simulink subsystem "Measurements"  (R2022a)
settings: Solver=VariableStepAuto  StartTime=0.0  StopTime=10.0  RelTol=1e-3
undefined symbols (not defined in the file): D0, D1, D13, D3, D6, PTA1, PTC16, PTC17, PTC2, PTD1
libraries: frdmk64flib x5
settings Model: Creator=bkfre  LastModifiedBy=bkfre

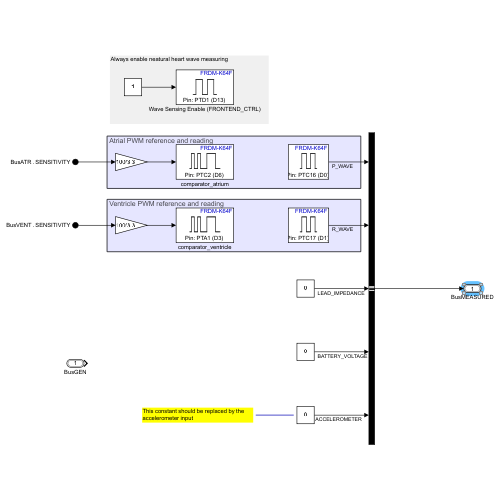
[thumbnail: Simulink's stored preview of the top-level diagram]
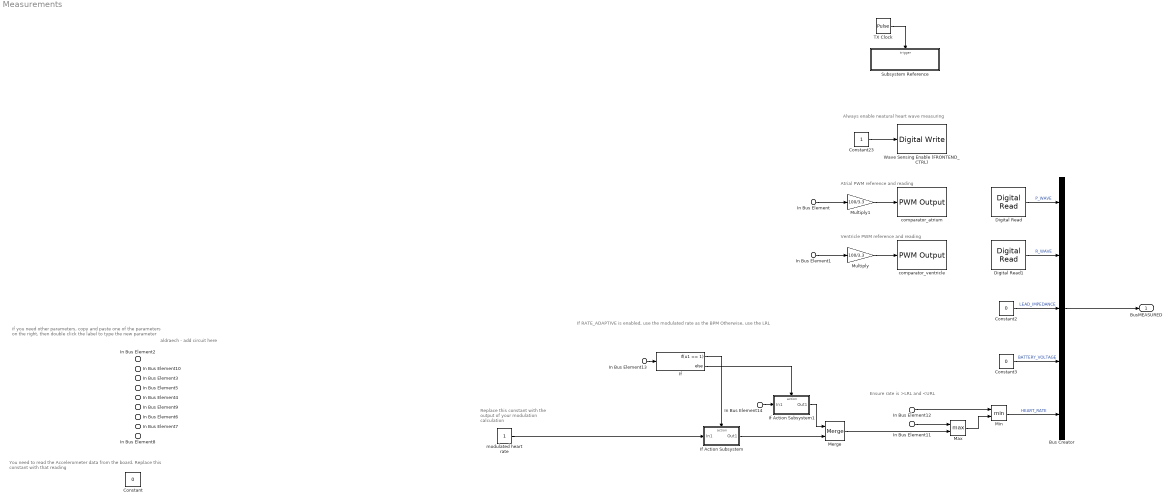
== system Measurements ==
  note: If RATE_ADAPTIVE is enabled, use the modulated rate as the BPM
      | Otherwise, use the LRL
  note: Replace this constant with the output of your modulation calculation
  note: Always enable neatural heart wave measuring
  note: Ventricle PWM reference and reading
  note: Atrial PWM reference and reading
  note: aldraech - add circuit here
  note: You need to read the Accelerometer data from the board. Replace this constant with that reading
  note: Ensure rate is >LRL and <URL
  note: if you need other parameters, copy and paste one of the parameters on the right, then double click the label to type the new parameter
  In Bus Element : Inport  PortName=BusATR  Element=SENSITIVITY
  In Bus Element1 : Inport  Port=2  PortName=BusVENT  Element=SENSITIVITY
  In Bus Element2 : Inport  Port=3  PortName=BusGEN  Element=LRL
  In Bus Element11 : Inport  Port=3  PortName=BusGEN  Element=LRL
  In Bus Element14 : Inport  Port=3  PortName=BusGEN  Element=LRL
  In Bus Element8 : Inport  Port=3  PortName=BusGEN  Element=URL
  In Bus Element12 : Inport  Port=3  PortName=BusGEN  Element=URL
  In Bus Element6 : Inport  Port=3  PortName=BusGEN  Element=MAX_SENSOR_RATE
  In Bus Element7 : Inport  Port=3  PortName=BusGEN  Element=RATE_SMOOTHING
  In Bus Element4 : Inport  Port=3  PortName=BusGEN  Element=ACTIVITY_THRESH
  In Bus Element3 : Inport  Port=3  PortName=BusGEN  Element=REACTION_TIME
  In Bus Element5 : Inport  Port=3  PortName=BusGEN  Element=RESPONSE_FACTOR
  In Bus Element9 : Inport  Port=3  PortName=BusGEN  Element=RESPONSE_FACTOR
  In Bus Element10 : Inport  Port=3  PortName=BusGEN  Element=RECOVERY_TIME
  In Bus Element13 : Inport  Port=3  PortName=BusGEN  Element=RATE_ADAPTIVE
  Bus Creator : BusCreator  Inputs=5  OutDataTypeStr=Bus: BusMEASURED  NonVirtualBus=on
  Constant : Constant  Value=0  OutDataTypeStr=double
  Constant2 : Constant  Value=0
  Constant23 : Constant  SampleTime=-1
  Constant3 : Constant  Value=0
  Digital Read : frdmk64flib/Digital Read  Whichpin=PTC16 (D0)  SampleTime=-1
  Digital Read1 : frdmk64flib/Digital Read  Whichpin=PTC17 (D1)  SampleTime=-1
  If : If  IfExpression=u1 == 1
  If Action Subsystem : Subsystem  TreatAsAtomicUnit=on
  If Action Subsystem1 : Subsystem  TreatAsAtomicUnit=on
  Max : MinMax  Function=max  Inputs=2
  Merge : Merge
  Min : MinMax  Inputs=2
  Multiply : Gain  Gain=100/3.3
  Multiply1 : Gain  Gain=100/3.3
  Subsystem Reference : Subsystem  ReferencedSubsystem=SerialTX
  TX Clock : DiscretePulseGenerator  PulseType=Time based  Period=0.1  PulseWidth=50
  Wave Sensing Enable (FRONTEND_CTRL) : frdmk64flib/Digital Write  Whichpin=PTD1 (D13)
  comparator_atrium : frdmk64flib/PWM Output  Whichpin=PTC2 (D6)  InitialFrequency=2000  InitialDutyCycle=0
  comparator_ventricle : frdmk64flib/PWM Output  Whichpin=PTA1 (D3)  InitialFrequency=2000  InitialDutyCycle=0
  modulated heart rate : Constant
  BusMEASURED : Outport  OutDataTypeStr=Bus: BusMEASURED
  wires:
  Constant2/1 -> Bus Creator/3  "LEAD_IMPEDANCE"
  Digital Read/1 -> Bus Creator/1  "P_WAVE"
  Digital Read1/1 -> Bus Creator/2  "R_WAVE"
  Constant3/1 -> Bus Creator/4  "BATTERY_VOLTAGE"
  Bus Creator/1 -> BusMEASURED/1
  Min/1 -> Bus Creator/5  "HEART_RATE"
  Constant23/1 -> Wave Sensing Enable (FRONTEND_CTRL)/1
  Multiply/1 -> comparator_ventricle/1
  In Bus Element1/1 -> Multiply/1
  Multiply1/1 -> comparator_atrium/1
  In Bus Element/1 -> Multiply1/1
  Max/1 -> Min/2
  In Bus Element12/1 -> Min/1
  In Bus Element11/1 -> Max/1
  modulated heart rate/1 -> If Action Subsystem/1(In1)
  In Bus Element13/1 -> If/1
  If/2 -> If Action Subsystem1/Action
  If/1 -> If Action Subsystem/Action
  In Bus Element14/1 -> If Action Subsystem1/1(In1)
  If Action Subsystem1/1(Out1) -> Merge/1
  Merge/1 -> Max/2
  If Action Subsystem/1(Out1) -> Merge/2
  TX Clock/1 -> Subsystem Reference/Trigger

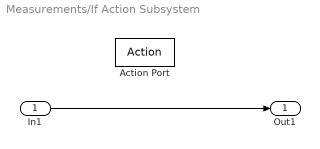
== system Measurements/If Action Subsystem ==
  In1 : Inport
  Action Port : ActionPort
  Out1 : Outport
  wires:
  In1/1 -> Out1/1

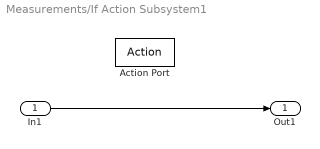
== system Measurements/If Action Subsystem1 ==
  In1 : Inport
  Action Port : ActionPort
  Out1 : Outport
  wires:
  In1/1 -> Out1/1
